simulink model "DatosAleatoriosR16"  (R2023b)
settings: Solver=ode45  StartTime=0.0  StopTime=7  RelTol=1e-3  EnableMultiTasking=on
libraries: simulink x1
settings Model: Creator=Helbert  LastModifiedBy=mluser
settings SolverCC: AlgebraicLoopSolver=TrustRegion
settings DataIOCC: LimitDataPoints=on  SaveFormat=Array  SignalLoggingSaveFormat=ModelDataLogs  ReturnWorkspaceOutputs=off
settings OptimizationCC: InitFltsAndDblsToZero=on  LifeSpan=inf
settings DebuggingCC: SaveWithParameterizedLinksMsg=none  UnderspecifiedInitializationDetection=Classic  MergeDetectMultiDrivingBlocksExec=none  SignalResolutionControl=TryResolveAllWithWarning  SolverPrmCheckMsg=warning  MultiTaskDSMMsg=warning  MultiTaskCondExecSysMsg=none  UnconnectedInputMsg=warning  UnconnectedOutputMsg=warning  UnconnectedLineMsg=warning  SFUnexpectedBacktrackingDiag=warning  SFNoUnconditionalDefaultTransitionDiag=warning  SFExecutionAtInitializationDiag=none  ArithmeticOperatorsInVariantConditions=warning
settings HardwareCC: ProdBitPerPointer=32  ProdBitPerSizeT=32  ProdBitPerPtrDiffT=32  ProdLargestAtomicFloat=None  ProdIntDivRoundTo=Undefined  ProdEndianess=Unspecified  ProdWordSize=32  ProdHWDeviceType=32-bit Generic
settings ModelReferenceCC: EnableRefExpFcnMdlSchedulingChecks=on  PropagateSignalLabelsOutOfModel=off
settings SFSimCC: SimUseLocalCustomCode=off  CustomCodeUndefinedFunction=UseInterfaceOnly
settings RTWCC: RTWUseLocalCustomCode=off
settings CodeAppCC: StateflowObjectComments=on
settings GRTTargetCC: TargetFcnLib=ansi_tfl_tmw.mat  TargetLangStandard=C89/C90 (ANSI)  CombineOutputUpdateFcns=off  GRTInterface=on
settings ConfigComp: CovMetricSettings=dw  CovSaveCumulativeToWorkspaceVar=on  CovSaveSingleToWorkspaceVar=on  CovExternalEMLEnable=off

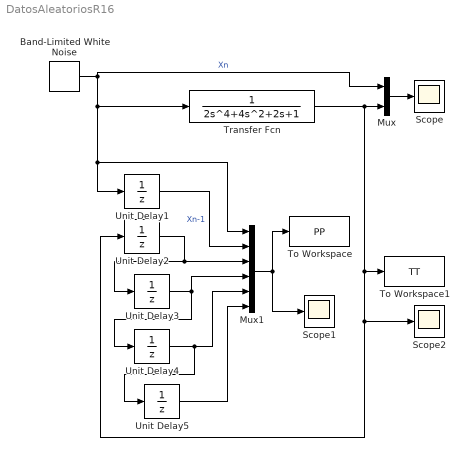
== system DatosAleatoriosR16 ==
  Band-Limited White Noise : simulink/Sources/Band-Limited White Noise  Cov=[15]  Ts=2  seed=[23341]
  Mux : Mux  Inputs=2
  Mux1 : Mux  Inputs=6
  Scope : Scope
  Scope1 : Scope
  Scope2 : Scope
  To Workspace : ToWorkspace  VariableName=PP  SampleTime=0.1
  To Workspace1 : ToWorkspace  VariableName=TT  SampleTime=0.1
  Transfer Fcn : TransferFcn  Denominator=[2 0 4 2 1]  ContinuousStateAttributes=0
  Unit Delay{1..5} (5 alike) : UnitDelay  SampleTime=0.1  HasFrameUpgradeWarning=on
  wires:
  Transfer Fcn/1 -> Mux/2, Scope2/1, Unit Delay2/1, To Workspace1/1
  Mux/1 -> Scope/1
  Band-Limited White Noise/1 -> Mux/1, Mux1/1, Unit Delay1/1, Transfer Fcn/1  "Xn"
  Unit Delay2/1 -> Unit Delay3/1, Mux1/3
  Mux1/1 -> To Workspace/1, Scope1/1
  Unit Delay1/1 -> Mux1/2  "Xn-1"
  Unit Delay3/1 -> Unit Delay4/1, Mux1/4
  Unit Delay4/1 -> Unit Delay5/1, Mux1/5
  Unit Delay5/1 -> Mux1/6
